simulink model "estimator_test"  (R2018b)
settings: Solver=FixedStepAuto  StartTime=0.0  StopTime=12000  FixedStep=simParams.sample_time_s  RelTol=1e-3  EnableMultiTasking=on
undefined symbols (not defined in the file or in its folder): actuators_lib, Actuators_Lib, DiscIntNeverNeededParam, Environment_lib, FSW_Lib, fswParams, gyro_body_radps, gyro_meas_valid, mag_body_T, mag_meas_valid, photodiodes_A, satelliteDynamics_lib, Sensors_Lib, simParams, solar_panel_power_W, sunsensor_body_deg, sunsensor_valid
libraries: gyroscope_lib x3, magnetometer_lib x3, rwa_assembly_torqueinput_lib x1, gravityGrad_Lib x1, atmoDrag_lib x1, magField_lib x1, solarPressure_lib x1, clock_lib x1, time_Lib x1, MEKF_LibraryR2018b x1, solar_panels_lib x1, sun_sensor_lib x1
settings Model: Creator=devantormey  LastModifiedBy=devantormey
settings OptimizationCC: LifeSpan=inf
settings DebuggingCC: SFUnexpectedBacktrackingDiag=warning  SFNoUnconditionalDefaultTransitionDiag=warning
settings SFSimCC: SimUseLocalCustomCode=off
settings RTWCC: RTWUseLocalCustomCode=off
settings CodeAppCC: StateflowObjectComments=on
settings GRTTargetCC: TargetLangStandard=C89/C90 (ANSI)  GeneratePreprocessorConditionals=Disable all
settings ConfigComp: CovMetricSettings=dw  CovHtmlReporting=on  CovSaveCumulativeToWorkspaceVar=on  CovSaveSingleToWorkspaceVar=on  CovExternalEMLEnable=off

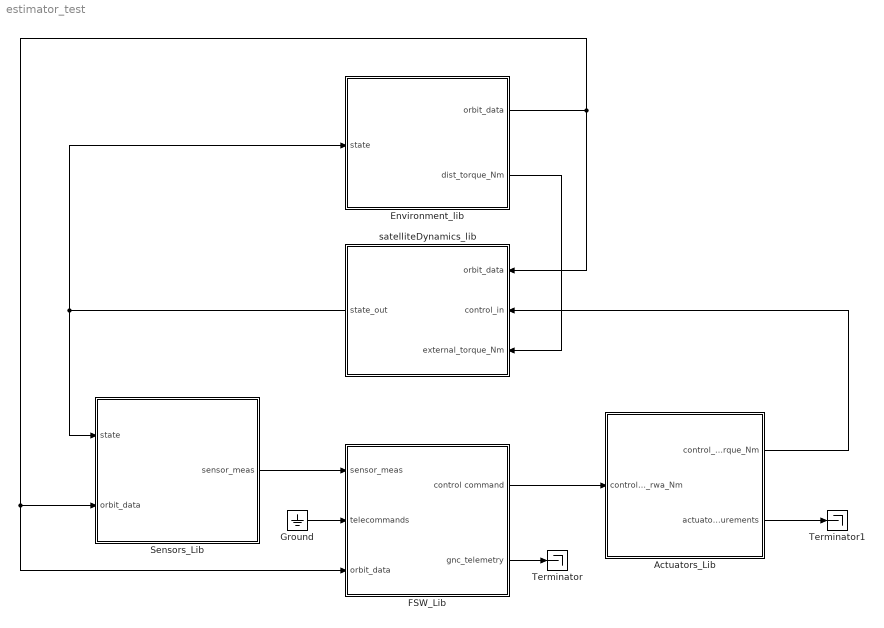
== system estimator_test ==
  Actuators_Lib : Subsystem  AncestorBlock=actuators_lib/Actuators_Lib
  Environment_lib : Subsystem  AncestorBlock=Environment_lib/Environment_lib
  FSW_Lib : Subsystem  AncestorBlock=FSW_Lib/FSW_Lib
  Ground : Ground
  Sensors_Lib : Subsystem  AncestorBlock=Sensors_Lib/Sensors_Lib
  Terminator : Terminator
  Terminator1 : Terminator
  satelliteDynamics_lib : Subsystem  AncestorBlock=satelliteDynamics_lib/satelliteDynamics_lib
  wires:
  FSW_Lib/1(control command) -> Actuators_Lib/1(control_cmd_rwa_Nm)
  Actuators_Lib/1(control_torque_Nm) -> satelliteDynamics_lib/2(control_in)
  satelliteDynamics_lib/1(state_out) -> Environment_lib/1(state), Sensors_Lib/1(state)
  Sensors_Lib/1(sensor_meas) -> FSW_Lib/1(sensor_meas)
  Actuators_Lib/2(actuator_measurements) -> Terminator1/1
  Ground/1 -> FSW_Lib/2(telecommands)
  Environment_lib/1(orbit_data) -> FSW_Lib/3(orbit_data), Sensors_Lib/2(orbit_data), satelliteDynamics_lib/1(orbit_data)
  Environment_lib/2(dist_torque_Nm) -> satelliteDynamics_lib/3(external_torque_Nm)
  FSW_Lib/2(gnc_telemetry) -> Terminator/1

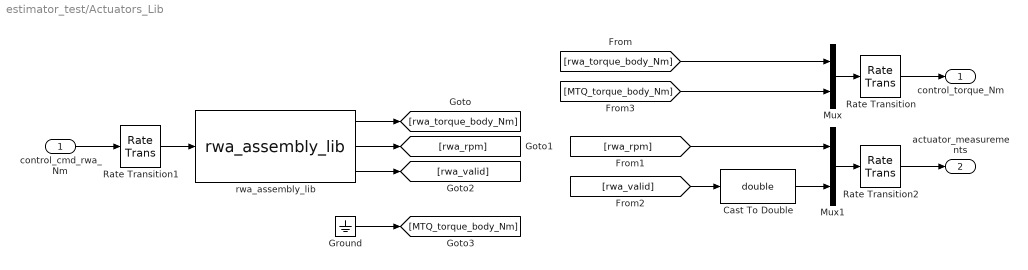
== system estimator_test/Actuators_Lib ==
  control_cmd_rwa_Nm : Inport
  Cast To Double : DataTypeConversion  OutDataTypeStr=double
  Ground : Ground
  Mux : Mux  Inputs=[3 3]
  Mux1 : Mux  Inputs=[4 4]
  Rate Transition : RateTransition
  Rate Transition1 : RateTransition  OutPortSampleTime=simParams.actuators.sample_time_s
  Rate Transition2 : RateTransition
  rwa_assembly_lib : rwa_assembly_torqueinput_lib/rwa_assembly_lib  SystemSampleTime=-1
  control_torque_Nm : Outport
  actuator_measurements : Outport  Port=2
  wires:
  Cast To Double/1 -> Mux1/2
  Rate Transition2/1 -> actuator_measurements/1
  Ground/1 -> [MTQ_torque_body_Nm]
  Mux/1 -> Rate Transition/1
  [rwa_torque_body_Nm] -> Mux/1
  [MTQ_torque_body_Nm] -> Mux/2
  Rate Transition1/1 -> rwa_assembly_lib/1
  Mux1/1 -> Rate Transition2/1
  [rwa_valid] -> Cast To Double/1
  [rwa_rpm] -> Mux1/1
  rwa_assembly_lib/1 -> [rwa_torque_body_Nm]
  rwa_assembly_lib/3 -> [rwa_valid]
  rwa_assembly_lib/2 -> [rwa_rpm]
  control_cmd_rwa_Nm/1 -> Rate Transition1/1
  Rate Transition/1 -> control_torque_Nm/1

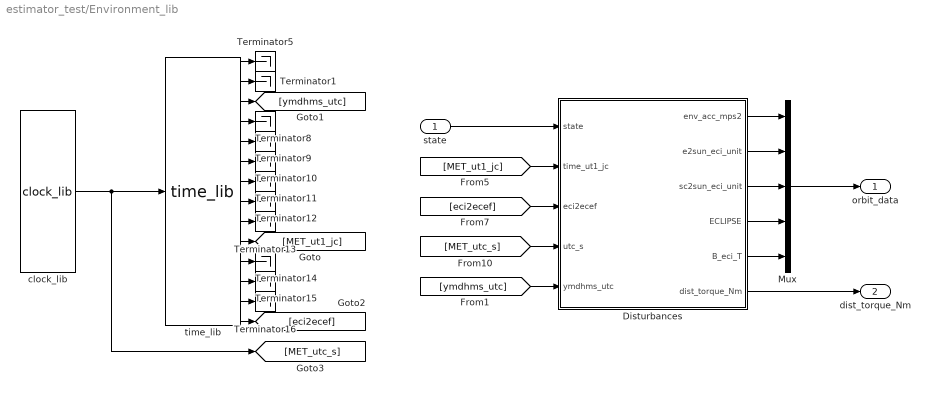
== system estimator_test/Environment_lib ==
  state : Inport
  Disturbances : Subsystem
  Mux : Mux  Inputs=[3 3 3 1 3]
  Terminator{1,5,8..16} (11 alike) : Terminator
  clock_lib : clock_lib/clock_lib  SystemSampleTime=-1
  "time_lib " : time_Lib/time_lib    SystemSampleTime=-1
  orbit_data : Outport
  dist_torque_Nm : Outport  Port=2
  wires:
  state/1 -> Disturbances/1(state)
  Disturbances/1(env_acc_mps2) -> Mux/1
  Disturbances/4(ECLIPSE) -> Mux/4
  "time_lib "/9 -> Terminator13/1
  [ymdhms_utc] -> Disturbances/5(ymdhms_utc)
  "time_lib "/7 -> Terminator11/1
  "time_lib "/11 -> Terminator14/1
  "time_lib "/8 -> Terminator12/1
  "time_lib "/1 -> Terminator5/1
  Disturbances/6(dist_torque_Nm) -> dist_torque_Nm/1
  clock_lib/1 -> "time_lib "/1, [MET_utc_s]
  Mux/1 -> orbit_data/1
  "time_lib "/5 -> Terminator9/1
  "time_lib "/14 -> [eci2ecef]
  [eci2ecef] -> Disturbances/3(eci2ecef)
  "time_lib "/3 -> [ymdhms_utc]
  "time_lib "/6 -> Terminator10/1
  "time_lib "/12 -> Terminator15/1
  Disturbances/3(sc2sun_eci_unit) -> Mux/3
  [MET_ut1_jc] -> Disturbances/2(time_ut1_jc)
  "time_lib "/2 -> Terminator1/1
  "time_lib "/13 -> Terminator16/1
  "time_lib "/4 -> Terminator8/1
  Disturbances/2(e2sun_eci_unit) -> Mux/2
  Disturbances/5(B_eci_T) -> Mux/5
  [MET_utc_s] -> Disturbances/4(utc_s)
  "time_lib "/10 -> [MET_ut1_jc]

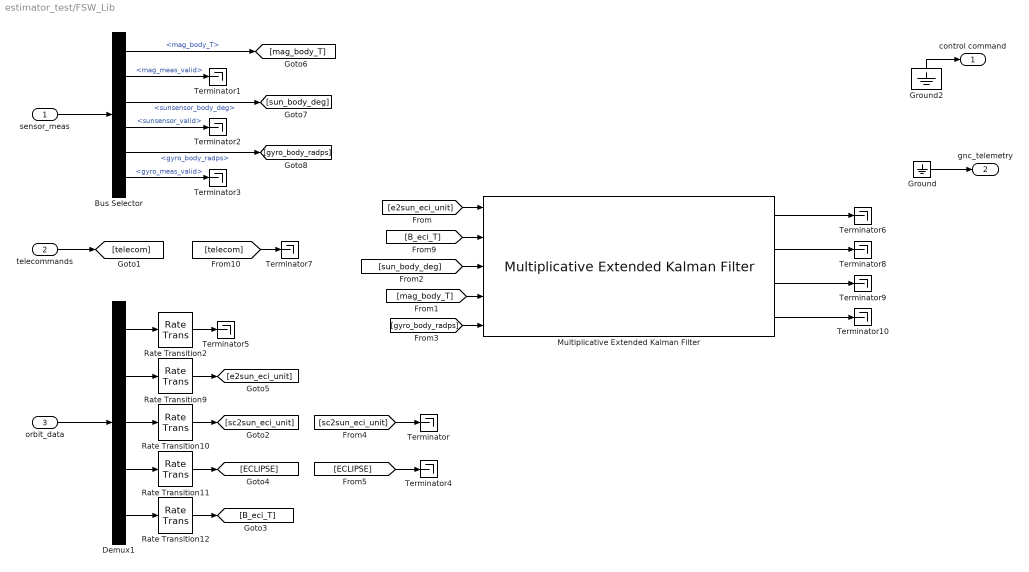
== system estimator_test/FSW_Lib ==
  sensor_meas : Inport
  telecommands : Inport  Port=2
  orbit_data : Inport  Port=3
  Bus Selector : BusSelector  OutputSignals=mag_body_T,mag_meas_valid,sunsensor_body_deg,sunsensor_valid,gyro_body_radps,gyro_meas_valid
  Demux1 : Demux  Outputs=[3 3 3 1 3]
  Ground : Ground
  Ground2 : Ground
  Multiplicative Extended Kalman Filter : MEKF_LibraryR2018b/Multiplicative Extended Kalman Filter  SystemSampleTime=-1
  Rate Transition{2,9..12} (5 alike) : RateTransition  OutPortSampleTime=simParams.sensors.sample_time_s
  Terminator{,1..10} (11 alike) : Terminator
  control command : Outport
  gnc_telemetry : Outport  Port=2
  wires:
  [telecom] -> Terminator7/1
  [B_eci_T] -> Multiplicative Extended Kalman Filter/2
  [e2sun_eci_unit] -> Multiplicative Extended Kalman Filter/1
  Demux1/4 -> Rate Transition11/1
  Rate Transition2/1 -> Terminator5/1
  Demux1/5 -> Rate Transition12/1
  Rate Transition9/1 -> [e2sun_eci_unit]
  Rate Transition10/1 -> [sc2sun_eci_unit]
  Demux1/3 -> Rate Transition10/1
  Rate Transition12/1 -> [B_eci_T]
  Demux1/1 -> Rate Transition2/1
  Rate Transition11/1 -> [ECLIPSE]
  Demux1/2 -> Rate Transition9/1
  orbit_data/1 -> Demux1/1
  Ground2/1 -> control command/1
  Ground/1 -> gnc_telemetry/1
  telecommands/1 -> [telecom]
  sensor_meas/1 -> Bus Selector/1
  [sun_body_deg] -> Multiplicative Extended Kalman Filter/3
  Bus Selector/1 -> [mag_body_T]  "<mag_body_T>"
  [mag_body_T] -> Multiplicative Extended Kalman Filter/4
  Bus Selector/3 -> [sun_body_deg]  "<sunsensor_body_deg>"
  Bus Selector/2 -> Terminator1/1  "<mag_meas_valid>"
  Bus Selector/4 -> Terminator2/1  "<sunsensor_valid>"
  Bus Selector/5 -> [gyro_body_radps]  "<gyro_body_radps>"
  [gyro_body_radps] -> Multiplicative Extended Kalman Filter/5
  Bus Selector/6 -> Terminator3/1  "<gyro_meas_valid>"
  [sc2sun_eci_unit] -> Terminator/1
  [ECLIPSE] -> Terminator4/1
  Multiplicative Extended Kalman Filter/1 -> Terminator6/1
  Multiplicative Extended Kalman Filter/2 -> Terminator8/1
  Multiplicative Extended Kalman Filter/3 -> Terminator9/1
  Multiplicative Extended Kalman Filter/4 -> Terminator10/1

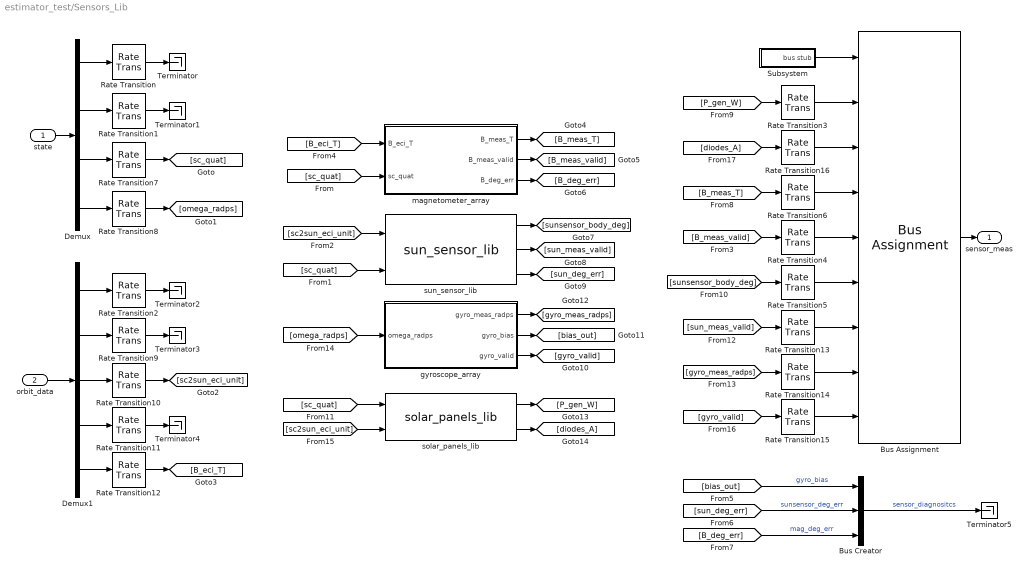
== system estimator_test/Sensors_Lib ==
  state : Inport
  orbit_data : Inport  Port=2
  Bus Assignment : BusAssignment  AssignedSignals=solar_panel_power_W,photodiodes_A,mag_body_T,mag_meas_valid,sunsensor_body_deg,sunsensor_valid,gyro_body_radps,gyro_meas_valid
  Bus Creator : BusCreator  Inputs=3
  Demux : Demux  Outputs=[3 3 4 3]
  Demux1 : Demux  Outputs=[3 3 3 1 3]
  Rate Transition{,1..16} (17 alike) : RateTransition  OutPortSampleTime=simParams.sensors.sample_time_s
  Subsystem : Subsystem
  Terminator{,1..5} (6 alike) : Terminator
  gyroscope_array : Subsystem
  magnetometer_array : Subsystem
  solar_panels_lib : solar_panels_lib/solar_panels_lib  SystemSampleTime=-1
  "sun_sensor_lib " : sun_sensor_lib/sun_sensor_lib   SystemSampleTime=-1
  sensor_meas : Outport
  wires:
  [diodes_A] -> Rate Transition16/1
  Rate Transition16/1 -> Bus Assignment/3
  Rate Transition3/1 -> Bus Assignment/2
  Rate Transition6/1 -> Bus Assignment/4
  Rate Transition4/1 -> Bus Assignment/5
  Rate Transition5/1 -> Bus Assignment/6
  Rate Transition13/1 -> Bus Assignment/7
  Rate Transition14/1 -> Bus Assignment/8
  Rate Transition15/1 -> Bus Assignment/9
  solar_panels_lib/2 -> [diodes_A]
  Bus Creator/1 -> Terminator5/1  "sensor_diagnositcs"
  [B_deg_err] -> Bus Creator/3  "mag_deg_err"
  [sun_deg_err] -> Bus Creator/2  "sunsensor_deg_err"
  [bias_out] -> Bus Creator/1  "gyro_bias"
  [gyro_valid] -> Rate Transition15/1
  [gyro_meas_radps] -> Rate Transition14/1
  [sun_meas_valid] -> Rate Transition13/1
  [sunsensor_body_deg] -> Rate Transition5/1
  [B_meas_valid] -> Rate Transition4/1
  [P_gen_W] -> Rate Transition3/1
  [B_meas_T] -> Rate Transition6/1
  solar_panels_lib/1 -> [P_gen_W]
  [sc_quat] -> solar_panels_lib/1
  [sc2sun_eci_unit] -> solar_panels_lib/2
  Demux1/1 -> Rate Transition2/1
  Rate Transition2/1 -> Terminator2/1
  Rate Transition9/1 -> Terminator3/1
  Demux1/2 -> Rate Transition9/1
  Rate Transition10/1 -> [sc2sun_eci_unit]
  Demux1/3 -> Rate Transition10/1
  Rate Transition11/1 -> Terminator4/1
  Demux1/4 -> Rate Transition11/1
  Rate Transition12/1 -> [B_eci_T]
  Demux1/5 -> Rate Transition12/1
  Rate Transition/1 -> Terminator/1
  Demux/1 -> Rate Transition/1
  Rate Transition1/1 -> Terminator1/1
  Demux/2 -> Rate Transition1/1
  Rate Transition7/1 -> [sc_quat]
  Demux/3 -> Rate Transition7/1
  Demux/4 -> Rate Transition8/1
  Rate Transition8/1 -> [omega_radps]
  gyroscope_array/3(gyro_valid) -> [gyro_valid]
  gyroscope_array/2(gyro_bias) -> [bias_out]
  gyroscope_array/1(gyro_meas_radps) -> [gyro_meas_radps]
  "sun_sensor_lib "/3 -> [sun_deg_err]
  "sun_sensor_lib "/2 -> [sun_meas_valid]
  "sun_sensor_lib "/1 -> [sunsensor_body_deg]
  magnetometer_array/3(B_deg_err) -> [B_deg_err]
  magnetometer_array/2(B_meas_valid) -> [B_meas_valid]
  magnetometer_array/1(B_meas_T) -> [B_meas_T]
  Subsystem/1(bus stub) -> Bus Assignment/1
  [B_eci_T] -> magnetometer_array/1(B_eci_T)
  [sc2sun_eci_unit] -> "sun_sensor_lib "/1
  orbit_data/1 -> Demux1/1
  [omega_radps] -> gyroscope_array/1(omega_radps)
  [sc_quat] -> "sun_sensor_lib "/2
  [sc_quat] -> magnetometer_array/2(sc_quat)
  state/1 -> Demux/1
  Bus Assignment/1 -> sensor_meas/1

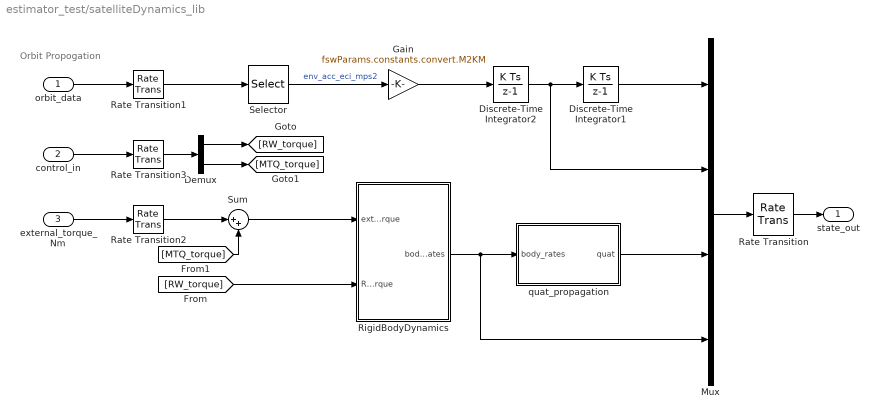
== system estimator_test/satelliteDynamics_lib ==
  note: Orbit Propogation
  orbit_data : Inport
  control_in : Inport  Port=2
  external_torque_Nm : Inport  Port=3
  Demux : Demux  Outputs=[3 3]
  Discrete-Time Integrator1 : DiscreteIntegrator  InitialCondition=simParams.initialConditions.r0  SampleTime=-1  ICPrevOutput=DiscIntNeverNeededParam  ICPrevScaledInput=DiscIntNeverNeededParam
  Discrete-Time Integrator2 : DiscreteIntegrator  InitialCondition=simParams.initialConditions.v0  SampleTime=-1  ICPrevOutput=DiscIntNeverNeededParam  ICPrevScaledInput=DiscIntNeverNeededParam
  Gain : Gain  Gain=fswParams.constants.convert.M2KM
  Mux : Mux  Inputs=[3 3 4 3]
  Rate Transition : RateTransition  InitialCondition=[simParams.initialConditions.r0;simParams.initialConditions.v0;simParams.initialConditions.q0;simParams.initialConditions.w0]
  Rate Transition1 : RateTransition  OutPortSampleTime=simParams.sample_time_s
  Rate Transition2 : RateTransition  OutPortSampleTime=simParams.sample_time_s
  Rate Transition3 : RateTransition  OutPortSampleTime=simParams.sample_time_s
  RigidBodyDynamics : Subsystem
  Selector : Selector  InputPortWidth=13  IndexOptions=Index vector (dialog)  Indices=[1 2 3]  OutputSizes=1
  Sum : Sum  Inputs=|++
  quat_propagation : Subsystem
  state_out : Outport
  wires:
  Sum/1 -> RigidBodyDynamics/1(external_torque)
  [MTQ_torque] -> Sum/2
  [RW_torque] -> RigidBodyDynamics/2(RW_torque)
  Demux/2 -> [MTQ_torque]
  Demux/1 -> [RW_torque]
  Rate Transition3/1 -> Demux/1
  Rate Transition2/1 -> Sum/1
  RigidBodyDynamics/1(body_rates) -> quat_propagation/1(body_rates), Mux/4
  quat_propagation/1(quat) -> Mux/3
  Selector/1 -> Gain/1  "env_acc_eci_mps2"
  external_torque_Nm/1 -> Rate Transition2/1
  Rate Transition1/1 -> Selector/1
  orbit_data/1 -> Rate Transition1/1
  Rate Transition/1 -> state_out/1
  Gain/1 -> Discrete-Time Integrator2/1
  Discrete-Time Integrator1/1 -> Mux/1
  Discrete-Time Integrator2/1 -> Discrete-Time Integrator1/1, Mux/2
  Mux/1 -> Rate Transition/1
  control_in/1 -> Rate Transition3/1

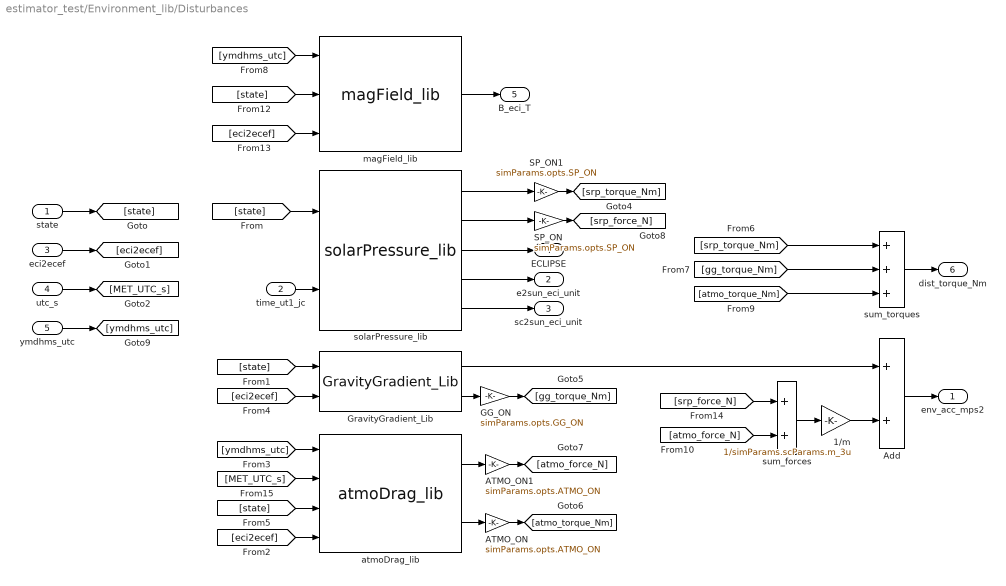
== system estimator_test/Environment_lib/Disturbances ==
  state : Inport
  time_ut1_jc : Inport  Port=2
  eci2ecef : Inport  Port=3
  utc_s : Inport  Port=4
  ymdhms_utc : Inport  Port=5
  1/m : Gain  Gain=1/simParams.scParams.m_3u
  ATMO_ON : Gain  Gain=simParams.opts.ATMO_ON
  ATMO_ON1 : Gain  Gain=simParams.opts.ATMO_ON
  Add : Sum
  GG_ON : Gain  Gain=simParams.opts.GG_ON
  "GravityGradient_Lib " : gravityGrad_Lib/GravityGradient_Lib   SystemSampleTime=-1
  SP_ON : Gain  Gain=simParams.opts.SP_ON
  "SP_ON1 " : Gain  Gain=simParams.opts.SP_ON
  atmoDrag_lib : atmoDrag_lib/atmoDrag_lib  SystemSampleTime=-1
  magField_lib : magField_lib/magField_lib  SystemSampleTime=-1
      link override Rate Transition2: InitialCondition=0
  solarPressure_lib : solarPressure_lib/solarPressure_lib  SystemSampleTime=-1
  sum_forces : Sum
  sum_torques : Sum  Inputs=+++
  env_acc_mps2 : Outport
  e2sun_eci_unit : Outport  Port=2
  sc2sun_eci_unit : Outport  Port=3
  ECLIPSE : Outport  Port=4
  B_eci_T : Outport  Port=5
  dist_torque_Nm : Outport  Port=6
  wires:
  solarPressure_lib/5 -> sc2sun_eci_unit/1
  magField_lib/1 -> B_eci_T/1
  [eci2ecef] -> magField_lib/3
  [ymdhms_utc] -> magField_lib/1
  ymdhms_utc/1 -> [ymdhms_utc]
  [state] -> magField_lib/2
  "GravityGradient_Lib "/2 -> GG_ON/1
  "GravityGradient_Lib "/1 -> Add/1
  SP_ON/1 -> [srp_force_N]
  ATMO_ON1/1 -> [atmo_force_N]
  [srp_force_N] -> sum_forces/1
  [atmo_force_N] -> sum_forces/2
  [atmo_torque_Nm] -> sum_torques/3
  sum_torques/1 -> dist_torque_Nm/1
  [eci2ecef] -> "GravityGradient_Lib "/2
  [gg_torque_Nm] -> sum_torques/2
  GG_ON/1 -> [gg_torque_Nm]
  [srp_torque_Nm] -> sum_torques/1
  "SP_ON1 "/1 -> [srp_torque_Nm]
  [MET_UTC_s] -> atmoDrag_lib/2
  [ymdhms_utc] -> atmoDrag_lib/1
  utc_s/1 -> [MET_UTC_s]
  [state] -> atmoDrag_lib/3
  [eci2ecef] -> atmoDrag_lib/4
  eci2ecef/1 -> [eci2ecef]
  [state] -> "GravityGradient_Lib "/1
  [state] -> solarPressure_lib/1
  state/1 -> [state]
  ATMO_ON/1 -> [atmo_torque_Nm]
  atmoDrag_lib/1 -> ATMO_ON1/1
  atmoDrag_lib/2 -> ATMO_ON/1
  1/m/1 -> Add/2
  Add/1 -> env_acc_mps2/1
  sum_forces/1 -> 1/m/1
  time_ut1_jc/1 -> solarPressure_lib/2
  solarPressure_lib/2 -> SP_ON/1
  solarPressure_lib/4 -> e2sun_eci_unit/1
  solarPressure_lib/1 -> "SP_ON1 "/1
  solarPressure_lib/3 -> ECLIPSE/1

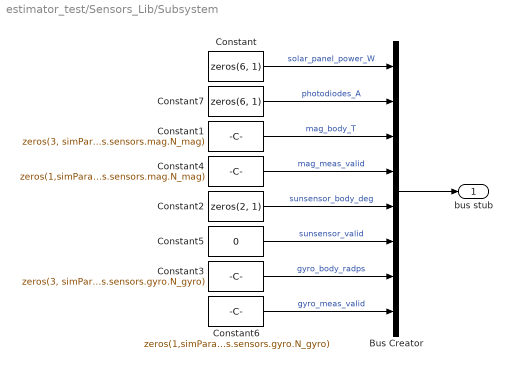
== system estimator_test/Sensors_Lib/Subsystem ==
  Bus Creator : BusCreator  Inputs=8
  Constant : Constant  Value=zeros(6, 1)
  Constant1 : Constant  Value=zeros(3, simParams.sensors.mag.N_mag)
  Constant2 : Constant  Value=zeros(2, 1)
  Constant3 : Constant  Value=zeros(3, simParams.sensors.gyro.N_gyro)
  Constant4 : Constant  Value=zeros(1,simParams.sensors.mag.N_mag)
  Constant5 : Constant  Value=0
  Constant6 : Constant  Value=zeros(1,simParams.sensors.gyro.N_gyro)
  Constant7 : Constant  Value=zeros(6, 1)
  bus stub : Outport
  wires:
  Constant7/1 -> Bus Creator/2  "photodiodes_A"
  Constant6/1 -> Bus Creator/8  "gyro_meas_valid"
  Constant5/1 -> Bus Creator/6  "sunsensor_valid"
  Constant4/1 -> Bus Creator/4  "mag_meas_valid"
  Constant3/1 -> Bus Creator/7  "gyro_body_radps"
  Bus Creator/1 -> bus stub/1
  Constant2/1 -> Bus Creator/5  "sunsensor_body_deg"
  Constant1/1 -> Bus Creator/3  "mag_body_T"
  Constant/1 -> Bus Creator/1  "solar_panel_power_W"

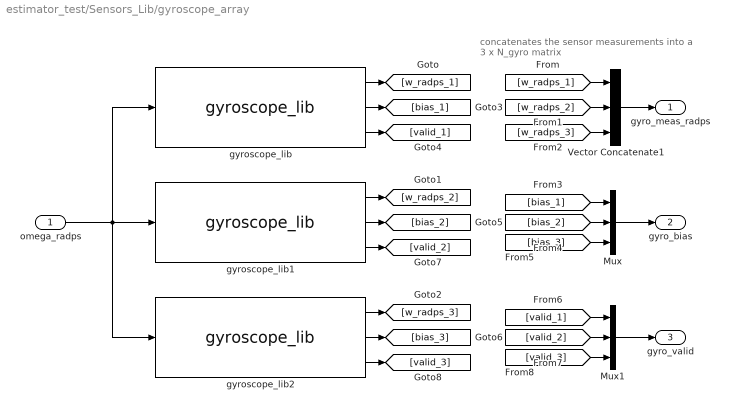
== system estimator_test/Sensors_Lib/gyroscope_array ==
  note: concatenates the sensor measurements
      | into a 3 x N_gyro matrix
  omega_radps : Inport
  Mux : Mux  Inputs=3
  Mux1 : Mux  Inputs=3
  Vector Concatenate1 : Concatenate  NumInputs=3  Mode=Multidimensional array  ConcatenateDimension=2
  gyroscope_lib : gyroscope_lib/gyroscope_lib  id_s=1
  gyroscope_lib1 : gyroscope_lib/gyroscope_lib  id_s=2
  gyroscope_lib2 : gyroscope_lib/gyroscope_lib  id_s=3
  gyro_meas_radps : Outport
  gyro_bias : Outport  Port=2
  gyro_valid : Outport  Port=3
  wires:
  [valid_3] -> Mux1/3
  [valid_2] -> Mux1/2
  [valid_1] -> Mux1/1
  Mux1/1 -> gyro_valid/1
  [bias_3] -> Mux/3
  [bias_2] -> Mux/2
  [bias_1] -> Mux/1
  Mux/1 -> gyro_bias/1
  [w_radps_3] -> Vector Concatenate1/3
  [w_radps_2] -> Vector Concatenate1/2
  [w_radps_1] -> Vector Concatenate1/1
  Vector Concatenate1/1 -> gyro_meas_radps/1
  gyroscope_lib2/3 -> [valid_3]
  gyroscope_lib1/3 -> [valid_2]
  gyroscope_lib2/2 -> [bias_3]
  gyroscope_lib1/2 -> [bias_2]
  gyroscope_lib/3 -> [valid_1]
  gyroscope_lib/2 -> [bias_1]
  gyroscope_lib2/1 -> [w_radps_3]
  gyroscope_lib1/1 -> [w_radps_2]
  gyroscope_lib/1 -> [w_radps_1]
  omega_radps/1 -> gyroscope_lib1/1, gyroscope_lib/1, gyroscope_lib2/1

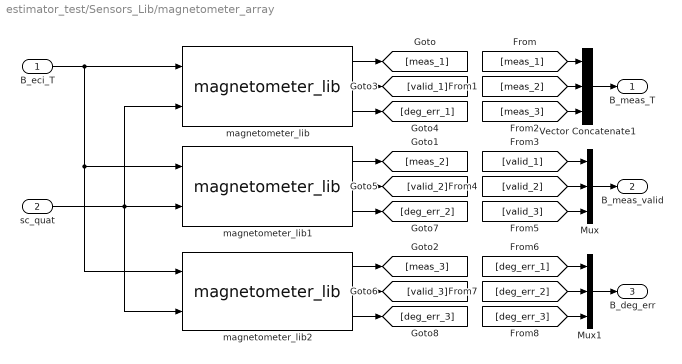
== system estimator_test/Sensors_Lib/magnetometer_array ==
  B_eci_T : Inport
  sc_quat : Inport  Port=2
  Mux : Mux  Inputs=3
  Mux1 : Mux  Inputs=3
  Vector Concatenate1 : Concatenate  NumInputs=3  Mode=Multidimensional array  ConcatenateDimension=2
  magnetometer_lib : magnetometer_lib/magnetometer_lib  id_s=1
  magnetometer_lib1 : magnetometer_lib/magnetometer_lib  id_s=2
  magnetometer_lib2 : magnetometer_lib/magnetometer_lib  id_s=1
  B_meas_T : Outport
  B_meas_valid : Outport  Port=2
  B_deg_err : Outport  Port=3
  wires:
  [deg_err_3] -> Mux1/3
  [deg_err_2] -> Mux1/2
  [deg_err_1] -> Mux1/1
  Mux1/1 -> B_deg_err/1
  [valid_3] -> Mux/3
  [valid_2] -> Mux/2
  [valid_1] -> Mux/1
  Mux/1 -> B_meas_valid/1
  [meas_3] -> Vector Concatenate1/3
  [meas_2] -> Vector Concatenate1/2
  [meas_1] -> Vector Concatenate1/1
  Vector Concatenate1/1 -> B_meas_T/1
  magnetometer_lib2/3 -> [deg_err_3]
  magnetometer_lib1/3 -> [deg_err_2]
  magnetometer_lib2/2 -> [valid_3]
  magnetometer_lib1/2 -> [valid_2]
  magnetometer_lib/3 -> [deg_err_1]
  magnetometer_lib/2 -> [valid_1]
  magnetometer_lib2/1 -> [meas_3]
  magnetometer_lib1/1 -> [meas_2]
  magnetometer_lib/1 -> [meas_1]
  B_eci_T/1 -> magnetometer_lib1/1, magnetometer_lib2/1, magnetometer_lib/1
  sc_quat/1 -> magnetometer_lib1/2, magnetometer_lib2/2, magnetometer_lib/2

== system estimator_test/satelliteDynamics_lib/RigidBodyDynamics ==
  external_torque : Inport
  RW_torque : Inport  Port=2
  Discrete-Time Integrator : DiscreteIntegrator  InitialCondition=[0;0;0]  SampleTime=-1  ICPrevOutput=DiscIntNeverNeededParam  ICPrevScaledInput=DiscIntNeverNeededParam
  "Discrete-Time Integrator " : DiscreteIntegrator  InitialCondition=simParams.initialConditions.w0  SampleTime=-1  ICPrevOutput=DiscIntNeverNeededParam  ICPrevScaledInput=DiscIntNeverNeededParam
  dynamics : Subsystem
  body_rates : Outport
  wires:
  dynamics/1(omega_dot) -> "Discrete-Time Integrator "/1
  external_torque/1 -> dynamics/1(external_torque_Nm)
  "Discrete-Time Integrator "/1 -> dynamics/4(omega_radps), body_rates/1
  Discrete-Time Integrator/1 -> dynamics/3(rw_momentum_Nms)
  RW_torque/1 -> Discrete-Time Integrator/1, dynamics/2(rw_torque_Nm)

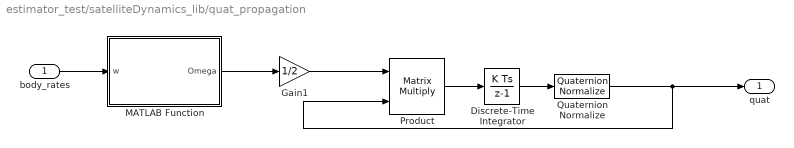
== system estimator_test/satelliteDynamics_lib/quat_propagation ==
  body_rates : Inport
  Discrete-Time Integrator : DiscreteIntegrator  InitialCondition=simParams.initialConditions.q0  SampleTime=-1  ICPrevOutput=DiscIntNeverNeededParam  ICPrevScaledInput=DiscIntNeverNeededParam
  Gain1 : Gain  Gain=1/2
  MATLAB Function : MATLAB Function  TreatAsAtomicUnit=on
  Product : Product  Multiplication=Matrix(*)  RndMeth=Zero
  Quaternion Normalize : sharedutil/Quaternion Normalize  aMode=aMode
      settings: SourceProductName=Aerospace Blockset  SourceProductBaseCode=AE
  quat : Outport
  wires:
  MATLAB Function/1(Omega) -> Gain1/1
  body_rates/1 -> MATLAB Function/1(w)
  Quaternion Normalize/1 -> Product/2, quat/1
  Gain1/1 -> Product/1
  Discrete-Time Integrator/1 -> Quaternion Normalize/1
  Product/1 -> Discrete-Time Integrator/1

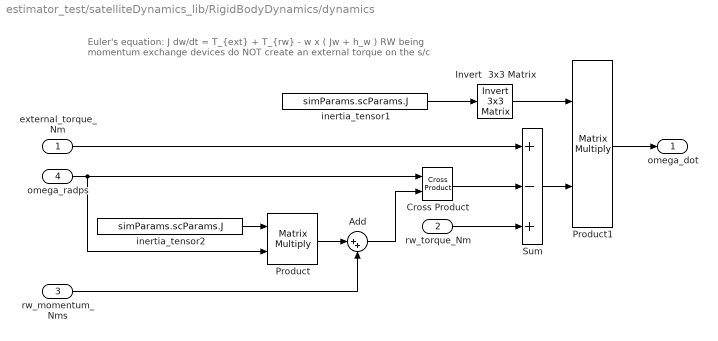
== system estimator_test/satelliteDynamics_lib/RigidBodyDynamics/dynamics ==
  note: Euler's equation: J dw/dt = T_{ext} + T_{rw} - w x ( Jw + h_w )
      |
      | RW being momentum exchange devices do NOT create
      | an external torque on the s/c
  external_torque_Nm : Inport
  rw_torque_Nm : Inport  Port=2
  rw_momentum_Nms : Inport  Port=3
  omega_radps : Inport  Port=4
  Add : Sum  Inputs=|++
  Cross Product : vrlib/Utilities/Cross Product
      settings: SourceProductBaseCode=VR
  Invert  3x3 Matrix : aerolibutil/Invert  3x3 Matrix
  Product : Product  Multiplication=Matrix(*)  RndMeth=Zero
  Product1 : Product  Multiplication=Matrix(*)  RndMeth=Zero
  Sum : Sum  Inputs=+-+
  inertia_tensor1 : Constant  Value=simParams.scParams.J
  inertia_tensor2 : Constant  Value=simParams.scParams.J
  omega_dot : Outport
  wires:
  rw_momentum_Nms/1 -> Add/2
  external_torque_Nm/1 -> Sum/1
  omega_radps/1 -> Product/2, Cross Product/1
  inertia_tensor2/1 -> Product/1
  Sum/1 -> Product1/2
  Product1/1 -> omega_dot/1
  Invert  3x3 Matrix/1 -> Product1/1
  inertia_tensor1/1 -> Invert  3x3 Matrix/1
  Cross Product/1 -> Sum/2
  Product/1 -> Add/1
  Add/1 -> Cross Product/2
  rw_torque_Nm/1 -> Sum/3

== matlab function estimator_test/satelliteDynamics_lib/quat_propagation/MATLAB Function ==
  data: w input; Omega output
function Omega = skew_sym(w)
%#codegen

    w_skew = ...
        [0 w(3) -w(2);
        -w(3) 0 w(1);
        w(2) -w(1) 0];

    Omega = ...
        [0 -w';
        w w_skew];
